simulink model "TSR_Scenario_002_cs"  (R2014b)
settings: Solver=ode5  SolverMode=SingleTasking  StartTime=0.0  StopTime=inf  FixedStep=1/100  RelTol=1e-3
PreLoadFcn:
  | mbxruntime.callbacks.PreLoadFcn(bdroot);
  | check_NUTS_defined;
  | 
  | assignin('base',['model_closed_' bdroot],false);
  | 
  | addpath('../includes_TSR/includes_TSR');
  | 
  | switch version('-release')
  | case {'2010a', '2010b', '2011a'}
  | addpath('../includes_TSR/ML2010b');
  | otherwise
  | addpath('../includes_TSR/ML2011b');
  | end
PostLoadFcn:
  | mbxruntime.callbacks.PostLoadFcn(bdroot);
InitFcn:
  | mbxruntime.callbacks.InitFcn(bdroot);;
  | 
  | addpath('..\includes_TSR');
StartFcn:
  | mbxruntime.callbacks.StartFcn(bdroot);
StopFcn:
  | mbxruntime.callbacks.StopFcn(bdroot);
model workspace: external: MAT-File .\TSR_Scenario_002_cs_hws.mat (data not in the file)
undefined symbols (not defined in the file or in its folder): InitImageOutputDir, mbxruntime, OrientationPitch, OrientationRoll, PositionX, PositionY, PositionZ, tabledata, warningInitialVelocity, x0
undefined symbols (not defined in the file): SteeringColumn, SteeringWheel, TSR_Scenario_002_cs_003e47b1b59594b6, TSR_Scenario_002_cs_023e87a31011dc74, TSR_Scenario_002_cs_048cb8409c90d9c6, TSR_Scenario_002_cs_106a0284aafa53e6, TSR_Scenario_002_cs_195b368d22a7f172, TSR_Scenario_002_cs_1e339fa5d680f213, TSR_Scenario_002_cs_26196a9fb104f950, TSR_Scenario_002_cs_261a709f6f453598, TSR_Scenario_002_cs_2ac3337370d0049d, TSR_Scenario_002_cs_2dc51e6a68b01b00, TSR_Scenario_002_cs_3460ff54d38ab2e2, TSR_Scenario_002_cs_42ea7d6e56bd6005, TSR_Scenario_002_cs_4dd419d6d2b56fc2, TSR_Scenario_002_cs_5316a21de09dff2f, TSR_Scenario_002_cs_538caacf3455966d, TSR_Scenario_002_cs_5b2cfdbcfc80811f, TSR_Scenario_002_cs_5ce0eafbb7a2dce7, TSR_Scenario_002_cs_62cdbf45c6f8824a, TSR_Scenario_002_cs_6bebc368eedff0bc, TSR_Scenario_002_cs_6d26481da4ed7e29, TSR_Scenario_002_cs_70c7e369ce6550e0, TSR_Scenario_002_cs_7a63051a1f311451, TSR_Scenario_002_cs_7d7dc8405f613c6d, TSR_Scenario_002_cs_7f65e296173485e8, TSR_Scenario_002_cs_87183cf6ff7bb4b6, TSR_Scenario_002_cs_8921b0da7ab80865, TSR_Scenario_002_cs_9495ce3a76763d1f, TSR_Scenario_002_cs_a679806a2fdc8099, TSR_Scenario_002_cs_Actros_1860_1_Path_pathUniqueID, TSR_Scenario_002_cs_Actros_2541_1_Path_pathUniqueID, TSR_Scenario_002_cs_Actros_2541_3_Path_pathUniqueID, TSR_Scenario_002_cs_Actros_2541_4_Path_pathUniqueID, TSR_Scenario_002_cs_adf24c93a9de8a4e, TSR_Scenario_002_cs_Audi_A8_1_Dynamics_Simple_initialPitch, TSR_Scenario_002_cs_Audi_A8_1_Dynamics_Simple_initialRoll, TSR_Scenario_002_cs_Audi_A8_1_Dynamics_Simple_initialX, TSR_Scenario_002_cs_Audi_A8_1_Dynamics_Simple_initialY, TSR_Scenario_002_cs_Audi_A8_1_Dynamics_Simple_initialYaw, TSR_Scenario_002_cs_Audi_A8_1_Dynamics_Simple_initialZ, TSR_Scenario_002_cs_b136c6ccb55f77db, TSR_Scenario_002_cs_ba4f809714c282b7, TSR_Scenario_002_cs_BMW_X5_1_Path_pathUniqueID, TSR_Scenario_002_cs_BMW_X5_1_SpeedProfile_speedProfileUniqueID, TSR_Scenario_002_cs_BMW_X5_2_Path_pathUniqueID, TSR_Scenario_002_cs_BMW_X5_2_SpeedProfile_speedProfileUniqueID, TSR_Scenario_002_cs_Citroen_C3_1_Path_pathUniqueID, TSR_Scenario_002_cs_Citroen_C3_2_Path_pathUniqueID, TSR_Scenario_002_cs_d8f275339b7082cf, TSR_Scenario_002_cs_Daf_95_1_Path_pathUniqueID, TSR_Scenario_002_cs_Daf_95_1_SpeedProfile_speedProfileUniqueID, TSR_Scenario_002_cs_dc019741510ce2f2, TSR_Scenario_002_cs_fdbc8aabe460b27c, TSR_Scenario_002_cs_Fiat_Bravo_1_Path_pathUniqueID, TSR_Scenario_002_cs_Ford_Fiesta_1_Path_pathUniqueID, TSR_Scenario_002_cs_Honda_Pan_European_1_Path_pathUniqueID, TSR_Scenario_002_cs_Mazda_RX8_1_Path_pathUniqueID, TSR_Scenario_002_cs_Nissan_Cabstar_1_Path_pathUniqueID, TSR_Scenario_002_cs_Nissan_Cabstar_2_Path_pathUniqueID ... (+9)
libraries: simulink_extras x82, simulink x23, PreScanSimulinkLibrary x11
(part 15 of 39)

== system TSR_Scenario_002_cs/VISUMatrixSign_HighwayOverhang_14 ==
  VISUMatrixSign_HighwayOverhang_14 : Inport  Tag=inport/VisuMatrixSign  SampleTime=1/100  BusOutputAsStruct=on
  Actuator : Subsystem  mask(PreScan Sink Block: VisuMatrixSign){UniqueID=1088, ResourceList={'1' 'InformationSign\MatrixSign_GreenArrow.png' '2' 'InformationSign\Empty.jpeg' '3' 'InformationSign\SEARCH_Logo.png' '4' 'InformationSign\z274-50_black_full.png' '5' 'InformationSign\z274-51_black_full.png' '6' 'InformationSign\z274-52_black_full.png' '7' 'InformationSign\z274-53_black_full.png' '8' 'InformationSign\z274-54_black_full.png' '9' 'InformationSign\z274-55_black_full.png' '10' 'InformationSign\z274-56_black_full.png' '11' 'InformationSign\z274-57_black_full.png' '12' 'InformationSign\z274-58_black_full.png' '13' 'InformationSign\z274-59_black_full.png' '14' 'InformationSign\z274-60_black_full.png' '15' 'InformationSign\z274-61_black_full.png' '16' 'InformationSign\z274-62_black_full.png' '17' 'InformationSign\z274-63_black_full.png' }, PivotName=}
      mask prompts: UniqueID "Parent Unique Identifier (auto-generated)"; ResourceList "Resource List (auto-generated)"; PivotName "Name of pivot (auto-generated)"
      mask help:
      | The VisuMatrixSign block provides a way to adapt the texture of the plates connected to an overhang, based on Resource IDs of the texture files.
      |
      | For more information, please click Help.
      mask Help: eval('openHelp(733)')
      mask Display: image(imread('HighwaySpeedMatrix.png'))
  wires:
  VISUMatrixSign_HighwayOverhang_14/1 -> Actuator/1(VISUMatrixSign_HighwayOverhang_14)

== system TSR_Scenario_002_cs/VISUMatrixSign_HighwayOverhang_15 ==
  VISUMatrixSign_HighwayOverhang_15 : Inport  Tag=inport/VisuMatrixSign  SampleTime=1/100  BusOutputAsStruct=on
  Actuator : Subsystem  mask(PreScan Sink Block: VisuMatrixSign){UniqueID=1090, ResourceList={'1' 'InformationSign\MatrixSign_GreenArrow.png' '2' 'InformationSign\Empty.jpeg' '3' 'InformationSign\SEARCH_Logo.png' '4' 'InformationSign\z274-50_black_full.png' '5' 'InformationSign\z274-51_black_full.png' '6' 'InformationSign\z274-52_black_full.png' '7' 'InformationSign\z274-53_black_full.png' '8' 'InformationSign\z274-54_black_full.png' '9' 'InformationSign\z274-55_black_full.png' '10' 'InformationSign\z274-56_black_full.png' '11' 'InformationSign\z274-57_black_full.png' '12' 'InformationSign\z274-58_black_full.png' '13' 'InformationSign\z274-59_black_full.png' '14' 'InformationSign\z274-60_black_full.png' '15' 'InformationSign\z274-61_black_full.png' '16' 'InformationSign\z274-62_black_full.png' '17' 'InformationSign\z274-63_black_full.png' }, PivotName=}
      mask prompts: UniqueID "Parent Unique Identifier (auto-generated)"; ResourceList "Resource List (auto-generated)"; PivotName "Name of pivot (auto-generated)"
      mask help:
      | The VisuMatrixSign block provides a way to adapt the texture of the plates connected to an overhang, based on Resource IDs of the texture files.
      |
      | For more information, please click Help.
      mask Help: eval('openHelp(733)')
      mask Display: image(imread('HighwaySpeedMatrix.png'))
  wires:
  VISUMatrixSign_HighwayOverhang_15/1 -> Actuator/1(VISUMatrixSign_HighwayOverhang_15)

== system TSR_Scenario_002_cs/VISUMatrixSign_HighwayOverhang_16 ==
  VISUMatrixSign_HighwayOverhang_16 : Inport  Tag=inport/VisuMatrixSign  SampleTime=1/100  BusOutputAsStruct=on
  Actuator : Subsystem  mask(PreScan Sink Block: VisuMatrixSign){UniqueID=1091, ResourceList={'1' 'InformationSign\MatrixSign_GreenArrow.png' '2' 'InformationSign\Empty.jpeg' '3' 'InformationSign\SEARCH_Logo.png' '4' 'InformationSign\z274-50_black_full.png' '5' 'InformationSign\z274-51_black_full.png' '6' 'InformationSign\z274-52_black_full.png' '7' 'InformationSign\z274-53_black_full.png' '8' 'InformationSign\z274-54_black_full.png' '9' 'InformationSign\z274-55_black_full.png' '10' 'InformationSign\z274-56_black_full.png' '11' 'InformationSign\z274-57_black_full.png' '12' 'InformationSign\z274-58_black_full.png' '13' 'InformationSign\z274-59_black_full.png' '14' 'InformationSign\z274-60_black_full.png' '15' 'InformationSign\z274-61_black_full.png' '16' 'InformationSign\z274-62_black_full.png' '17' 'InformationSign\z274-63_black_full.png' }, PivotName=}
      mask prompts: UniqueID "Parent Unique Identifier (auto-generated)"; ResourceList "Resource List (auto-generated)"; PivotName "Name of pivot (auto-generated)"
      mask help:
      | The VisuMatrixSign block provides a way to adapt the texture of the plates connected to an overhang, based on Resource IDs of the texture files.
      |
      | For more information, please click Help.
      mask Help: eval('openHelp(733)')
      mask Display: image(imread('HighwaySpeedMatrix.png'))
  wires:
  VISUMatrixSign_HighwayOverhang_16/1 -> Actuator/1(VISUMatrixSign_HighwayOverhang_16)

== system TSR_Scenario_002_cs/VISUMatrixSign_HighwayOverhang_17 ==
  VISUMatrixSign_HighwayOverhang_17 : Inport  Tag=inport/VisuMatrixSign  SampleTime=1/100  BusOutputAsStruct=on
  Actuator : Subsystem  mask(PreScan Sink Block: VisuMatrixSign){UniqueID=1092, ResourceList={'1' 'InformationSign\MatrixSign_GreenArrow.png' '2' 'InformationSign\Empty.jpeg' '3' 'InformationSign\SEARCH_Logo.png' '4' 'InformationSign\z274-50_black_full.png' '5' 'InformationSign\z274-51_black_full.png' '6' 'InformationSign\z274-52_black_full.png' '7' 'InformationSign\z274-53_black_full.png' '8' 'InformationSign\z274-54_black_full.png' '9' 'InformationSign\z274-55_black_full.png' '10' 'InformationSign\z274-56_black_full.png' '11' 'InformationSign\z274-57_black_full.png' '12' 'InformationSign\z274-58_black_full.png' '13' 'InformationSign\z274-59_black_full.png' '14' 'InformationSign\z274-60_black_full.png' '15' 'InformationSign\z274-61_black_full.png' '16' 'InformationSign\z274-62_black_full.png' '17' 'InformationSign\z274-63_black_full.png' }, PivotName=}
      mask prompts: UniqueID "Parent Unique Identifier (auto-generated)"; ResourceList "Resource List (auto-generated)"; PivotName "Name of pivot (auto-generated)"
      mask help:
      | The VisuMatrixSign block provides a way to adapt the texture of the plates connected to an overhang, based on Resource IDs of the texture files.
      |
      | For more information, please click Help.
      mask Help: eval('openHelp(733)')
      mask Display: image(imread('HighwaySpeedMatrix.png'))
  wires:
  VISUMatrixSign_HighwayOverhang_17/1 -> Actuator/1(VISUMatrixSign_HighwayOverhang_17)

== system TSR_Scenario_002_cs/VISUMatrixSign_HighwayOverhang_18 ==
  VISUMatrixSign_HighwayOverhang_18 : Inport  Tag=inport/VisuMatrixSign  SampleTime=1/100  BusOutputAsStruct=on
  Actuator : Subsystem  mask(PreScan Sink Block: VisuMatrixSign){UniqueID=1093, ResourceList={'1' 'InformationSign\MatrixSign_GreenArrow.png' '2' 'InformationSign\Empty.jpeg' '3' 'InformationSign\SEARCH_Logo.png' '4' 'InformationSign\z274-50_black_full.png' '5' 'InformationSign\z274-51_black_full.png' '6' 'InformationSign\z274-52_black_full.png' '7' 'InformationSign\z274-53_black_full.png' '8' 'InformationSign\z274-54_black_full.png' '9' 'InformationSign\z274-55_black_full.png' '10' 'InformationSign\z274-56_black_full.png' '11' 'InformationSign\z274-57_black_full.png' '12' 'InformationSign\z274-58_black_full.png' '13' 'InformationSign\z274-59_black_full.png' '14' 'InformationSign\z274-60_black_full.png' '15' 'InformationSign\z274-61_black_full.png' '16' 'InformationSign\z274-62_black_full.png' '17' 'InformationSign\z274-63_black_full.png' }, PivotName=}
      mask prompts: UniqueID "Parent Unique Identifier (auto-generated)"; ResourceList "Resource List (auto-generated)"; PivotName "Name of pivot (auto-generated)"
      mask help:
      | The VisuMatrixSign block provides a way to adapt the texture of the plates connected to an overhang, based on Resource IDs of the texture files.
      |
      | For more information, please click Help.
      mask Help: eval('openHelp(733)')
      mask Display: image(imread('HighwaySpeedMatrix.png'))
  wires:
  VISUMatrixSign_HighwayOverhang_18/1 -> Actuator/1(VISUMatrixSign_HighwayOverhang_18)

== system TSR_Scenario_002_cs/VISUMatrixSign_HighwayOverhang_19 ==
  VISUMatrixSign_HighwayOverhang_19 : Inport  Tag=inport/VisuMatrixSign  SampleTime=1/100  BusOutputAsStruct=on
  Actuator : Subsystem  mask(PreScan Sink Block: VisuMatrixSign){UniqueID=1095, ResourceList={'1' 'InformationSign\MatrixSign_GreenArrow.png' '2' 'InformationSign\Empty.jpeg' '3' 'InformationSign\SEARCH_Logo.png' '4' 'InformationSign\z274-50_black_full.png' '5' 'InformationSign\z274-51_black_full.png' '6' 'InformationSign\z274-52_black_full.png' '7' 'InformationSign\z274-53_black_full.png' '8' 'InformationSign\z274-54_black_full.png' '9' 'InformationSign\z274-55_black_full.png' '10' 'InformationSign\z274-56_black_full.png' '11' 'InformationSign\z274-57_black_full.png' '12' 'InformationSign\z274-58_black_full.png' '13' 'InformationSign\z274-59_black_full.png' '14' 'InformationSign\z274-60_black_full.png' '15' 'InformationSign\z274-61_black_full.png' '16' 'InformationSign\z274-62_black_full.png' '17' 'InformationSign\z274-63_black_full.png' }, PivotName=}
      mask prompts: UniqueID "Parent Unique Identifier (auto-generated)"; ResourceList "Resource List (auto-generated)"; PivotName "Name of pivot (auto-generated)"
      mask help:
      | The VisuMatrixSign block provides a way to adapt the texture of the plates connected to an overhang, based on Resource IDs of the texture files.
      |
      | For more information, please click Help.
      mask Help: eval('openHelp(733)')
      mask Display: image(imread('HighwaySpeedMatrix.png'))
  wires:
  VISUMatrixSign_HighwayOverhang_19/1 -> Actuator/1(VISUMatrixSign_HighwayOverhang_19)

== system TSR_Scenario_002_cs/VISUMatrixSign_HighwayOverhang_2 ==
  VISUMatrixSign_HighwayOverhang_2 : Inport  Tag=inport/VisuMatrixSign  SampleTime=1/100  BusOutputAsStruct=on
  Actuator : Subsystem  mask(PreScan Sink Block: VisuMatrixSign){UniqueID=432, ResourceList={'1' 'InformationSign\MatrixSign_GreenArrow.png' '2' 'InformationSign\Empty.jpeg' '3' 'InformationSign\SEARCH_Logo.png' '4' 'InformationSign\z274-50_black_full.png' '5' 'InformationSign\z274-51_black_full.png' '6' 'InformationSign\z274-52_black_full.png' '7' 'InformationSign\z274-53_black_full.png' '8' 'InformationSign\z274-54_black_full.png' '9' 'InformationSign\z274-55_black_full.png' '10' 'InformationSign\z274-56_black_full.png' '11' 'InformationSign\z274-57_black_full.png' '12' 'InformationSign\z274-58_black_full.png' '13' 'InformationSign\z274-59_black_full.png' '14' 'InformationSign\z274-60_black_full.png' '15' 'InformationSign\z274-61_black_full.png' '16' 'InformationSign\z274-62_black_full.png' '17' 'InformationSign\z274-63_black_full.png' }, PivotName=}
      mask prompts: UniqueID "Parent Unique Identifier (auto-generated)"; ResourceList "Resource List (auto-generated)"; PivotName "Name of pivot (auto-generated)"
      mask help:
      | The VisuMatrixSign block provides a way to adapt the texture of the plates connected to an overhang, based on Resource IDs of the texture files.
      |
      | For more information, please click Help.
      mask Help: eval('openHelp(733)')
      mask Display: image(imread('HighwaySpeedMatrix.png'))
  wires:
  VISUMatrixSign_HighwayOverhang_2/1 -> Actuator/1(VISUMatrixSign_HighwayOverhang_2)

== system TSR_Scenario_002_cs/VISUMatrixSign_HighwayOverhang_20 ==
  VISUMatrixSign_HighwayOverhang_20 : Inport  Tag=inport/VisuMatrixSign  SampleTime=1/100  BusOutputAsStruct=on
  Actuator : Subsystem  mask(PreScan Sink Block: VisuMatrixSign){UniqueID=1094, ResourceList={'1' 'InformationSign\MatrixSign_GreenArrow.png' '2' 'InformationSign\Empty.jpeg' '3' 'InformationSign\SEARCH_Logo.png' '4' 'InformationSign\z274-50_black_full.png' '5' 'InformationSign\z274-51_black_full.png' '6' 'InformationSign\z274-52_black_full.png' '7' 'InformationSign\z274-53_black_full.png' '8' 'InformationSign\z274-54_black_full.png' '9' 'InformationSign\z274-55_black_full.png' '10' 'InformationSign\z274-56_black_full.png' '11' 'InformationSign\z274-57_black_full.png' '12' 'InformationSign\z274-58_black_full.png' '13' 'InformationSign\z274-59_black_full.png' '14' 'InformationSign\z274-60_black_full.png' '15' 'InformationSign\z274-61_black_full.png' '16' 'InformationSign\z274-62_black_full.png' '17' 'InformationSign\z274-63_black_full.png' }, PivotName=}
      mask prompts: UniqueID "Parent Unique Identifier (auto-generated)"; ResourceList "Resource List (auto-generated)"; PivotName "Name of pivot (auto-generated)"
      mask help:
      | The VisuMatrixSign block provides a way to adapt the texture of the plates connected to an overhang, based on Resource IDs of the texture files.
      |
      | For more information, please click Help.
      mask Help: eval('openHelp(733)')
      mask Display: image(imread('HighwaySpeedMatrix.png'))
  wires:
  VISUMatrixSign_HighwayOverhang_20/1 -> Actuator/1(VISUMatrixSign_HighwayOverhang_20)

== system TSR_Scenario_002_cs/VISUMatrixSign_HighwayOverhang_21 ==
  VISUMatrixSign_HighwayOverhang_21 : Inport  Tag=inport/VisuMatrixSign  SampleTime=1/100  BusOutputAsStruct=on
  Actuator : Subsystem  mask(PreScan Sink Block: VisuMatrixSign){UniqueID=1099, ResourceList={'1' 'InformationSign\MatrixSign_GreenArrow.png' '2' 'InformationSign\Empty.jpeg' '3' 'InformationSign\SEARCH_Logo.png' '4' 'InformationSign\z274-50_black_full.png' '5' 'InformationSign\z274-51_black_full.png' '6' 'InformationSign\z274-52_black_full.png' '7' 'InformationSign\z274-53_black_full.png' '8' 'InformationSign\z274-54_black_full.png' '9' 'InformationSign\z274-55_black_full.png' '10' 'InformationSign\z274-56_black_full.png' '11' 'InformationSign\z274-57_black_full.png' '12' 'InformationSign\z274-58_black_full.png' '13' 'InformationSign\z274-59_black_full.png' '14' 'InformationSign\z274-60_black_full.png' '15' 'InformationSign\z274-61_black_full.png' '16' 'InformationSign\z274-62_black_full.png' '17' 'InformationSign\z274-63_black_full.png' }, PivotName=}
      mask prompts: UniqueID "Parent Unique Identifier (auto-generated)"; ResourceList "Resource List (auto-generated)"; PivotName "Name of pivot (auto-generated)"
      mask help:
      | The VisuMatrixSign block provides a way to adapt the texture of the plates connected to an overhang, based on Resource IDs of the texture files.
      |
      | For more information, please click Help.
      mask Help: eval('openHelp(733)')
      mask Display: image(imread('HighwaySpeedMatrix.png'))
  wires:
  VISUMatrixSign_HighwayOverhang_21/1 -> Actuator/1(VISUMatrixSign_HighwayOverhang_21)

== system TSR_Scenario_002_cs/VISUMatrixSign_HighwayOverhang_22 ==
  VISUMatrixSign_HighwayOverhang_22 : Inport  Tag=inport/VisuMatrixSign  SampleTime=1/100  BusOutputAsStruct=on
  Actuator : Subsystem  mask(PreScan Sink Block: VisuMatrixSign){UniqueID=1100, ResourceList={'1' 'InformationSign\MatrixSign_GreenArrow.png' '2' 'InformationSign\Empty.jpeg' '3' 'InformationSign\SEARCH_Logo.png' '4' 'InformationSign\z274-50_black_full.png' '5' 'InformationSign\z274-51_black_full.png' '6' 'InformationSign\z274-52_black_full.png' '7' 'InformationSign\z274-53_black_full.png' '8' 'InformationSign\z274-54_black_full.png' '9' 'InformationSign\z274-55_black_full.png' '10' 'InformationSign\z274-56_black_full.png' '11' 'InformationSign\z274-57_black_full.png' '12' 'InformationSign\z274-58_black_full.png' '13' 'InformationSign\z274-59_black_full.png' '14' 'InformationSign\z274-60_black_full.png' '15' 'InformationSign\z274-61_black_full.png' '16' 'InformationSign\z274-62_black_full.png' '17' 'InformationSign\z274-63_black_full.png' }, PivotName=}
      mask prompts: UniqueID "Parent Unique Identifier (auto-generated)"; ResourceList "Resource List (auto-generated)"; PivotName "Name of pivot (auto-generated)"
      mask help:
      | The VisuMatrixSign block provides a way to adapt the texture of the plates connected to an overhang, based on Resource IDs of the texture files.
      |
      | For more information, please click Help.
      mask Help: eval('openHelp(733)')
      mask Display: image(imread('HighwaySpeedMatrix.png'))
  wires:
  VISUMatrixSign_HighwayOverhang_22/1 -> Actuator/1(VISUMatrixSign_HighwayOverhang_22)

== system TSR_Scenario_002_cs/VISUMatrixSign_HighwayOverhang_23 ==
  VISUMatrixSign_HighwayOverhang_23 : Inport  Tag=inport/VisuMatrixSign  SampleTime=1/100  BusOutputAsStruct=on
  Actuator : Subsystem  mask(PreScan Sink Block: VisuMatrixSign){UniqueID=1102, ResourceList={'1' 'InformationSign\MatrixSign_GreenArrow.png' '2' 'InformationSign\Empty.jpeg' '3' 'InformationSign\SEARCH_Logo.png' '4' 'InformationSign\z274-50_black_full.png' '5' 'InformationSign\z274-51_black_full.png' '6' 'InformationSign\z274-52_black_full.png' '7' 'InformationSign\z274-53_black_full.png' '8' 'InformationSign\z274-54_black_full.png' '9' 'InformationSign\z274-55_black_full.png' '10' 'InformationSign\z274-56_black_full.png' '11' 'InformationSign\z274-57_black_full.png' '12' 'InformationSign\z274-58_black_full.png' '13' 'InformationSign\z274-59_black_full.png' '14' 'InformationSign\z274-60_black_full.png' '15' 'InformationSign\z274-61_black_full.png' '16' 'InformationSign\z274-62_black_full.png' '17' 'InformationSign\z274-63_black_full.png' }, PivotName=}
      mask prompts: UniqueID "Parent Unique Identifier (auto-generated)"; ResourceList "Resource List (auto-generated)"; PivotName "Name of pivot (auto-generated)"
      mask help:
      | The VisuMatrixSign block provides a way to adapt the texture of the plates connected to an overhang, based on Resource IDs of the texture files.
      |
      | For more information, please click Help.
      mask Help: eval('openHelp(733)')
      mask Display: image(imread('HighwaySpeedMatrix.png'))
  wires:
  VISUMatrixSign_HighwayOverhang_23/1 -> Actuator/1(VISUMatrixSign_HighwayOverhang_23)

== system TSR_Scenario_002_cs/VISUMatrixSign_HighwayOverhang_24 ==
  VISUMatrixSign_HighwayOverhang_24 : Inport  Tag=inport/VisuMatrixSign  SampleTime=1/100  BusOutputAsStruct=on
  Actuator : Subsystem  mask(PreScan Sink Block: VisuMatrixSign){UniqueID=1103, ResourceList={'1' 'InformationSign\MatrixSign_GreenArrow.png' '2' 'InformationSign\Empty.jpeg' '3' 'InformationSign\SEARCH_Logo.png' '4' 'InformationSign\z274-50_black_full.png' '5' 'InformationSign\z274-51_black_full.png' '6' 'InformationSign\z274-52_black_full.png' '7' 'InformationSign\z274-53_black_full.png' '8' 'InformationSign\z274-54_black_full.png' '9' 'InformationSign\z274-55_black_full.png' '10' 'InformationSign\z274-56_black_full.png' '11' 'InformationSign\z274-57_black_full.png' '12' 'InformationSign\z274-58_black_full.png' '13' 'InformationSign\z274-59_black_full.png' '14' 'InformationSign\z274-60_black_full.png' '15' 'InformationSign\z274-61_black_full.png' '16' 'InformationSign\z274-62_black_full.png' '17' 'InformationSign\z274-63_black_full.png' }, PivotName=}
      mask prompts: UniqueID "Parent Unique Identifier (auto-generated)"; ResourceList "Resource List (auto-generated)"; PivotName "Name of pivot (auto-generated)"
      mask help:
      | The VisuMatrixSign block provides a way to adapt the texture of the plates connected to an overhang, based on Resource IDs of the texture files.
      |
      | For more information, please click Help.
      mask Help: eval('openHelp(733)')
      mask Display: image(imread('HighwaySpeedMatrix.png'))
  wires:
  VISUMatrixSign_HighwayOverhang_24/1 -> Actuator/1(VISUMatrixSign_HighwayOverhang_24)

== system TSR_Scenario_002_cs/VISUMatrixSign_HighwayOverhang_25 ==
  VISUMatrixSign_HighwayOverhang_25 : Inport  Tag=inport/VisuMatrixSign  SampleTime=1/100  BusOutputAsStruct=on
  Actuator : Subsystem  mask(PreScan Sink Block: VisuMatrixSign){UniqueID=1104, ResourceList={'1' 'InformationSign\MatrixSign_GreenArrow.png' '2' 'InformationSign\Empty.jpeg' '3' 'InformationSign\SEARCH_Logo.png' '4' 'InformationSign\z274-50_black_full.png' '5' 'InformationSign\z274-51_black_full.png' '6' 'InformationSign\z274-52_black_full.png' '7' 'InformationSign\z274-53_black_full.png' '8' 'InformationSign\z274-54_black_full.png' '9' 'InformationSign\z274-55_black_full.png' '10' 'InformationSign\z274-56_black_full.png' '11' 'InformationSign\z274-57_black_full.png' '12' 'InformationSign\z274-58_black_full.png' '13' 'InformationSign\z274-59_black_full.png' '14' 'InformationSign\z274-60_black_full.png' '15' 'InformationSign\z274-61_black_full.png' '16' 'InformationSign\z274-62_black_full.png' '17' 'InformationSign\z274-63_black_full.png' }, PivotName=}
      mask prompts: UniqueID "Parent Unique Identifier (auto-generated)"; ResourceList "Resource List (auto-generated)"; PivotName "Name of pivot (auto-generated)"
      mask help:
      | The VisuMatrixSign block provides a way to adapt the texture of the plates connected to an overhang, based on Resource IDs of the texture files.
      |
      | For more information, please click Help.
      mask Help: eval('openHelp(733)')
      mask Display: image(imread('HighwaySpeedMatrix.png'))
  wires:
  VISUMatrixSign_HighwayOverhang_25/1 -> Actuator/1(VISUMatrixSign_HighwayOverhang_25)

== system TSR_Scenario_002_cs/VISUMatrixSign_HighwayOverhang_26 ==
  VISUMatrixSign_HighwayOverhang_26 : Inport  Tag=inport/VisuMatrixSign  SampleTime=1/100  BusOutputAsStruct=on
  Actuator : Subsystem  mask(PreScan Sink Block: VisuMatrixSign){UniqueID=1105, ResourceList={'1' 'InformationSign\MatrixSign_GreenArrow.png' '2' 'InformationSign\Empty.jpeg' '3' 'InformationSign\SEARCH_Logo.png' '4' 'InformationSign\z274-50_black_full.png' '5' 'InformationSign\z274-51_black_full.png' '6' 'InformationSign\z274-52_black_full.png' '7' 'InformationSign\z274-53_black_full.png' '8' 'InformationSign\z274-54_black_full.png' '9' 'InformationSign\z274-55_black_full.png' '10' 'InformationSign\z274-56_black_full.png' '11' 'InformationSign\z274-57_black_full.png' '12' 'InformationSign\z274-58_black_full.png' '13' 'InformationSign\z274-59_black_full.png' '14' 'InformationSign\z274-60_black_full.png' '15' 'InformationSign\z274-61_black_full.png' '16' 'InformationSign\z274-62_black_full.png' '17' 'InformationSign\z274-63_black_full.png' }, PivotName=}
      mask prompts: UniqueID "Parent Unique Identifier (auto-generated)"; ResourceList "Resource List (auto-generated)"; PivotName "Name of pivot (auto-generated)"
      mask help:
      | The VisuMatrixSign block provides a way to adapt the texture of the plates connected to an overhang, based on Resource IDs of the texture files.
      |
      | For more information, please click Help.
      mask Help: eval('openHelp(733)')
      mask Display: image(imread('HighwaySpeedMatrix.png'))
  wires:
  VISUMatrixSign_HighwayOverhang_26/1 -> Actuator/1(VISUMatrixSign_HighwayOverhang_26)

== system TSR_Scenario_002_cs/VISUMatrixSign_HighwayOverhang_27 ==
  VISUMatrixSign_HighwayOverhang_27 : Inport  Tag=inport/VisuMatrixSign  SampleTime=1/100  BusOutputAsStruct=on
  Actuator : Subsystem  mask(PreScan Sink Block: VisuMatrixSign){UniqueID=1106, ResourceList={'1' 'InformationSign\MatrixSign_GreenArrow.png' '2' 'InformationSign\Empty.jpeg' '3' 'InformationSign\SEARCH_Logo.png' '4' 'InformationSign\z274-50_black_full.png' '5' 'InformationSign\z274-51_black_full.png' '6' 'InformationSign\z274-52_black_full.png' '7' 'InformationSign\z274-53_black_full.png' '8' 'InformationSign\z274-54_black_full.png' '9' 'InformationSign\z274-55_black_full.png' '10' 'InformationSign\z274-56_black_full.png' '11' 'InformationSign\z274-57_black_full.png' '12' 'InformationSign\z274-58_black_full.png' '13' 'InformationSign\z274-59_black_full.png' '14' 'InformationSign\z274-60_black_full.png' '15' 'InformationSign\z274-61_black_full.png' '16' 'InformationSign\z274-62_black_full.png' '17' 'InformationSign\z274-63_black_full.png' }, PivotName=}
      mask prompts: UniqueID "Parent Unique Identifier (auto-generated)"; ResourceList "Resource List (auto-generated)"; PivotName "Name of pivot (auto-generated)"
      mask help:
      | The VisuMatrixSign block provides a way to adapt the texture of the plates connected to an overhang, based on Resource IDs of the texture files.
      |
      | For more information, please click Help.
      mask Help: eval('openHelp(733)')
      mask Display: image(imread('HighwaySpeedMatrix.png'))
  wires:
  VISUMatrixSign_HighwayOverhang_27/1 -> Actuator/1(VISUMatrixSign_HighwayOverhang_27)

== system TSR_Scenario_002_cs/VISUMatrixSign_HighwayOverhang_28 ==
  VISUMatrixSign_HighwayOverhang_28 : Inport  Tag=inport/VisuMatrixSign  SampleTime=1/100  BusOutputAsStruct=on
  Actuator : Subsystem  mask(PreScan Sink Block: VisuMatrixSign){UniqueID=1107, ResourceList={'1' 'InformationSign\MatrixSign_GreenArrow.png' '2' 'InformationSign\Empty.jpeg' '3' 'InformationSign\SEARCH_Logo.png' '4' 'InformationSign\z274-50_black_full.png' '5' 'InformationSign\z274-51_black_full.png' '6' 'InformationSign\z274-52_black_full.png' '7' 'InformationSign\z274-53_black_full.png' '8' 'InformationSign\z274-54_black_full.png' '9' 'InformationSign\z274-55_black_full.png' '10' 'InformationSign\z274-56_black_full.png' '11' 'InformationSign\z274-57_black_full.png' '12' 'InformationSign\z274-58_black_full.png' '13' 'InformationSign\z274-59_black_full.png' '14' 'InformationSign\z274-60_black_full.png' '15' 'InformationSign\z274-61_black_full.png' '16' 'InformationSign\z274-62_black_full.png' '17' 'InformationSign\z274-63_black_full.png' }, PivotName=}
      mask prompts: UniqueID "Parent Unique Identifier (auto-generated)"; ResourceList "Resource List (auto-generated)"; PivotName "Name of pivot (auto-generated)"
      mask help:
      | The VisuMatrixSign block provides a way to adapt the texture of the plates connected to an overhang, based on Resource IDs of the texture files.
      |
      | For more information, please click Help.
      mask Help: eval('openHelp(733)')
      mask Display: image(imread('HighwaySpeedMatrix.png'))
  wires:
  VISUMatrixSign_HighwayOverhang_28/1 -> Actuator/1(VISUMatrixSign_HighwayOverhang_28)

== system TSR_Scenario_002_cs/VISUMatrixSign_HighwayOverhang_3 ==
  VISUMatrixSign_HighwayOverhang_3 : Inport  Tag=inport/VisuMatrixSign  SampleTime=1/100  BusOutputAsStruct=on
  Actuator : Subsystem  mask(PreScan Sink Block: VisuMatrixSign){UniqueID=440, ResourceList={'1' 'InformationSign\MatrixSign_GreenArrow.png' '2' 'InformationSign\Empty.jpeg' '3' 'InformationSign\SEARCH_Logo.png' '4' 'InformationSign\z274-50_black_full.png' '5' 'InformationSign\z274-51_black_full.png' '6' 'InformationSign\z274-52_black_full.png' '7' 'InformationSign\z274-53_black_full.png' '8' 'InformationSign\z274-54_black_full.png' '9' 'InformationSign\z274-55_black_full.png' '10' 'InformationSign\z274-56_black_full.png' '11' 'InformationSign\z274-57_black_full.png' '12' 'InformationSign\z274-58_black_full.png' '13' 'InformationSign\z274-59_black_full.png' '14' 'InformationSign\z274-60_black_full.png' '15' 'InformationSign\z274-61_black_full.png' '16' 'InformationSign\z274-62_black_full.png' '17' 'InformationSign\z274-63_black_full.png' }, PivotName=}
      mask prompts: UniqueID "Parent Unique Identifier (auto-generated)"; ResourceList "Resource List (auto-generated)"; PivotName "Name of pivot (auto-generated)"
      mask help:
      | The VisuMatrixSign block provides a way to adapt the texture of the plates connected to an overhang, based on Resource IDs of the texture files.
      |
      | For more information, please click Help.
      mask Help: eval('openHelp(733)')
      mask Display: image(imread('HighwaySpeedMatrix.png'))
  wires:
  VISUMatrixSign_HighwayOverhang_3/1 -> Actuator/1(VISUMatrixSign_HighwayOverhang_3)

== system TSR_Scenario_002_cs/VISUMatrixSign_HighwayOverhang_4 ==
  VISUMatrixSign_HighwayOverhang_4 : Inport  Tag=inport/VisuMatrixSign  SampleTime=1/100  BusOutputAsStruct=on
  Actuator : Subsystem  mask(PreScan Sink Block: VisuMatrixSign){UniqueID=441, ResourceList={'1' 'InformationSign\MatrixSign_GreenArrow.png' '2' 'InformationSign\Empty.jpeg' '3' 'InformationSign\SEARCH_Logo.png' '4' 'InformationSign\z274-50_black_full.png' '5' 'InformationSign\z274-51_black_full.png' '6' 'InformationSign\z274-52_black_full.png' '7' 'InformationSign\z274-53_black_full.png' '8' 'InformationSign\z274-54_black_full.png' '9' 'InformationSign\z274-55_black_full.png' '10' 'InformationSign\z274-56_black_full.png' '11' 'InformationSign\z274-57_black_full.png' '12' 'InformationSign\z274-58_black_full.png' '13' 'InformationSign\z274-59_black_full.png' '14' 'InformationSign\z274-60_black_full.png' '15' 'InformationSign\z274-61_black_full.png' '16' 'InformationSign\z274-62_black_full.png' '17' 'InformationSign\z274-63_black_full.png' }, PivotName=}
      mask prompts: UniqueID "Parent Unique Identifier (auto-generated)"; ResourceList "Resource List (auto-generated)"; PivotName "Name of pivot (auto-generated)"
      mask help:
      | The VisuMatrixSign block provides a way to adapt the texture of the plates connected to an overhang, based on Resource IDs of the texture files.
      |
      | For more information, please click Help.
      mask Help: eval('openHelp(733)')
      mask Display: image(imread('HighwaySpeedMatrix.png'))
  wires:
  VISUMatrixSign_HighwayOverhang_4/1 -> Actuator/1(VISUMatrixSign_HighwayOverhang_4)

== system TSR_Scenario_002_cs/VISUMatrixSign_HighwayOverhang_5 ==
  VISUMatrixSign_HighwayOverhang_5 : Inport  Tag=inport/VisuMatrixSign  SampleTime=1/100  BusOutputAsStruct=on
  Actuator : Subsystem  mask(PreScan Sink Block: VisuMatrixSign){UniqueID=843, ResourceList={'1' 'InformationSign\MatrixSign_GreenArrow.png' '2' 'InformationSign\Empty.jpeg' '3' 'InformationSign\SEARCH_Logo.png' '4' 'InformationSign\z274-50_black_full.png' '5' 'InformationSign\z274-51_black_full.png' '6' 'InformationSign\z274-52_black_full.png' '7' 'InformationSign\z274-53_black_full.png' '8' 'InformationSign\z274-54_black_full.png' '9' 'InformationSign\z274-55_black_full.png' '10' 'InformationSign\z274-56_black_full.png' '11' 'InformationSign\z274-57_black_full.png' '12' 'InformationSign\z274-58_black_full.png' '13' 'InformationSign\z274-59_black_full.png' '14' 'InformationSign\z274-60_black_full.png' '15' 'InformationSign\z274-61_black_full.png' '16' 'InformationSign\z274-62_black_full.png' '17' 'InformationSign\z274-63_black_full.png' }, PivotName=}
      mask prompts: UniqueID "Parent Unique Identifier (auto-generated)"; ResourceList "Resource List (auto-generated)"; PivotName "Name of pivot (auto-generated)"
      mask help:
      | The VisuMatrixSign block provides a way to adapt the texture of the plates connected to an overhang, based on Resource IDs of the texture files.
      |
      | For more information, please click Help.
      mask Help: eval('openHelp(733)')
      mask Display: image(imread('HighwaySpeedMatrix.png'))
  wires:
  VISUMatrixSign_HighwayOverhang_5/1 -> Actuator/1(VISUMatrixSign_HighwayOverhang_5)

== system TSR_Scenario_002_cs/VISUMatrixSign_HighwayOverhang_6 ==
  VISUMatrixSign_HighwayOverhang_6 : Inport  Tag=inport/VisuMatrixSign  SampleTime=1/100  BusOutputAsStruct=on
  Actuator : Subsystem  mask(PreScan Sink Block: VisuMatrixSign){UniqueID=846, ResourceList={'1' 'InformationSign\MatrixSign_GreenArrow.png' '2' 'InformationSign\Empty.jpeg' '3' 'InformationSign\SEARCH_Logo.png' '4' 'InformationSign\z274-50_black_full.png' '5' 'InformationSign\z274-51_black_full.png' '6' 'InformationSign\z274-52_black_full.png' '7' 'InformationSign\z274-53_black_full.png' '8' 'InformationSign\z274-54_black_full.png' '9' 'InformationSign\z274-55_black_full.png' '10' 'InformationSign\z274-56_black_full.png' '11' 'InformationSign\z274-57_black_full.png' '12' 'InformationSign\z274-58_black_full.png' '13' 'InformationSign\z274-59_black_full.png' '14' 'InformationSign\z274-60_black_full.png' '15' 'InformationSign\z274-61_black_full.png' '16' 'InformationSign\z274-62_black_full.png' '17' 'InformationSign\z274-63_black_full.png' }, PivotName=}
      mask prompts: UniqueID "Parent Unique Identifier (auto-generated)"; ResourceList "Resource List (auto-generated)"; PivotName "Name of pivot (auto-generated)"
      mask help:
      | The VisuMatrixSign block provides a way to adapt the texture of the plates connected to an overhang, based on Resource IDs of the texture files.
      |
      | For more information, please click Help.
      mask Help: eval('openHelp(733)')
      mask Display: image(imread('HighwaySpeedMatrix.png'))
  wires:
  VISUMatrixSign_HighwayOverhang_6/1 -> Actuator/1(VISUMatrixSign_HighwayOverhang_6)

== system TSR_Scenario_002_cs/VISUMatrixSign_HighwayOverhang_7 ==
  VISUMatrixSign_HighwayOverhang_7 : Inport  Tag=inport/VisuMatrixSign  SampleTime=1/100  BusOutputAsStruct=on
  Actuator : Subsystem  mask(PreScan Sink Block: VisuMatrixSign){UniqueID=867, ResourceList={'1' 'InformationSign\MatrixSign_GreenArrow.png' '2' 'InformationSign\Empty.jpeg' '3' 'InformationSign\SEARCH_Logo.png' '4' 'InformationSign\z274-50_black_full.png' '5' 'InformationSign\z274-51_black_full.png' '6' 'InformationSign\z274-52_black_full.png' '7' 'InformationSign\z274-53_black_full.png' '8' 'InformationSign\z274-54_black_full.png' '9' 'InformationSign\z274-55_black_full.png' '10' 'InformationSign\z274-56_black_full.png' '11' 'InformationSign\z274-57_black_full.png' '12' 'InformationSign\z274-58_black_full.png' '13' 'InformationSign\z274-59_black_full.png' '14' 'InformationSign\z274-60_black_full.png' '15' 'InformationSign\z274-61_black_full.png' '16' 'InformationSign\z274-62_black_full.png' '17' 'InformationSign\z274-63_black_full.png' }, PivotName=}
      mask prompts: UniqueID "Parent Unique Identifier (auto-generated)"; ResourceList "Resource List (auto-generated)"; PivotName "Name of pivot (auto-generated)"
      mask help:
      | The VisuMatrixSign block provides a way to adapt the texture of the plates connected to an overhang, based on Resource IDs of the texture files.
      |
      | For more information, please click Help.
      mask Help: eval('openHelp(733)')
      mask Display: image(imread('HighwaySpeedMatrix.png'))
  wires:
  VISUMatrixSign_HighwayOverhang_7/1 -> Actuator/1(VISUMatrixSign_HighwayOverhang_7)

== system TSR_Scenario_002_cs/VISUMatrixSign_HighwayOverhang_8 ==
  VISUMatrixSign_HighwayOverhang_8 : Inport  Tag=inport/VisuMatrixSign  SampleTime=1/100  BusOutputAsStruct=on
  Actuator : Subsystem  mask(PreScan Sink Block: VisuMatrixSign){UniqueID=870, ResourceList={'1' 'InformationSign\MatrixSign_GreenArrow.png' '2' 'InformationSign\Empty.jpeg' '3' 'InformationSign\SEARCH_Logo.png' '4' 'InformationSign\z274-50_black_full.png' '5' 'InformationSign\z274-51_black_full.png' '6' 'InformationSign\z274-52_black_full.png' '7' 'InformationSign\z274-53_black_full.png' '8' 'InformationSign\z274-54_black_full.png' '9' 'InformationSign\z274-55_black_full.png' '10' 'InformationSign\z274-56_black_full.png' '11' 'InformationSign\z274-57_black_full.png' '12' 'InformationSign\z274-58_black_full.png' '13' 'InformationSign\z274-59_black_full.png' '14' 'InformationSign\z274-60_black_full.png' '15' 'InformationSign\z274-61_black_full.png' '16' 'InformationSign\z274-62_black_full.png' '17' 'InformationSign\z274-63_black_full.png' }, PivotName=}
      mask prompts: UniqueID "Parent Unique Identifier (auto-generated)"; ResourceList "Resource List (auto-generated)"; PivotName "Name of pivot (auto-generated)"
      mask help:
      | The VisuMatrixSign block provides a way to adapt the texture of the plates connected to an overhang, based on Resource IDs of the texture files.
      |
      | For more information, please click Help.
      mask Help: eval('openHelp(733)')
      mask Display: image(imread('HighwaySpeedMatrix.png'))
  wires:
  VISUMatrixSign_HighwayOverhang_8/1 -> Actuator/1(VISUMatrixSign_HighwayOverhang_8)

== system TSR_Scenario_002_cs/VISUMatrixSign_HighwayOverhang_9 ==
  VISUMatrixSign_HighwayOverhang_9 : Inport  Tag=inport/VisuMatrixSign  SampleTime=1/100  BusOutputAsStruct=on
  Actuator : Subsystem  mask(PreScan Sink Block: VisuMatrixSign){UniqueID=875, ResourceList={'1' 'InformationSign\MatrixSign_GreenArrow.png' '2' 'InformationSign\Empty.jpeg' '3' 'InformationSign\SEARCH_Logo.png' '4' 'InformationSign\z274-50_black_full.png' '5' 'InformationSign\z274-51_black_full.png' '6' 'InformationSign\z274-52_black_full.png' '7' 'InformationSign\z274-53_black_full.png' '8' 'InformationSign\z274-54_black_full.png' '9' 'InformationSign\z274-55_black_full.png' '10' 'InformationSign\z274-56_black_full.png' '11' 'InformationSign\z274-57_black_full.png' '12' 'InformationSign\z274-58_black_full.png' '13' 'InformationSign\z274-59_black_full.png' '14' 'InformationSign\z274-60_black_full.png' '15' 'InformationSign\z274-61_black_full.png' '16' 'InformationSign\z274-62_black_full.png' '17' 'InformationSign\z274-63_black_full.png' }, PivotName=}
      mask prompts: UniqueID "Parent Unique Identifier (auto-generated)"; ResourceList "Resource List (auto-generated)"; PivotName "Name of pivot (auto-generated)"
      mask help:
      | The VisuMatrixSign block provides a way to adapt the texture of the plates connected to an overhang, based on Resource IDs of the texture files.
      |
      | For more information, please click Help.
      mask Help: eval('openHelp(733)')
      mask Display: image(imread('HighwaySpeedMatrix.png'))
  wires:
  VISUMatrixSign_HighwayOverhang_9/1 -> Actuator/1(VISUMatrixSign_HighwayOverhang_9)

== system TSR_Scenario_002_cs/WheelL0_Audi_A8_1 ==
  WheelL0_Audi_A8_1 : Inport  Tag=inport/JointActuator  OutDataTypeStr=Bus: PRESCAN_POSE_DATA  SampleTime=1/100  BusOutputAsStruct=on
  Actuator : Subsystem  Tag=VisuJoint  mask(PreScan Sink Block: VisuJoint){UniqueID=13, Translate_ObjectID3D=Audi_A8_1.WheelL0, Rotate_ObjectID3D=Audi_A8_1.WheelL0, TimeStep=1/100, DisplayName=[]}
      mask prompts: UniqueID "Parent Unique ID"; Translate_ObjectID3D "Translate Object Name"; Rotate_ObjectID3D "Rotate Object Name"; TimeStep "Simulation Step"; DisplayName "Display Name"
      mask help:
      | The VisuJoint block provides a way to adapt the location and orientation of a part of an object.
      |
      | For more information, please click Help.
      settings: DeleteFcn=PreScanBlockDeleteFcn;
      mask Help: eval('openHelp(223)')
      mask Display: image(imread('Joint.png'))
  wires:
  WheelL0_Audi_A8_1/1 -> Actuator/1(Joint)

== system TSR_Scenario_002_cs/WheelL0_BMW_X5_2 ==
  WheelL0_BMW_X5_2 : Inport  Tag=inport/JointActuator  OutDataTypeStr=Bus: PRESCAN_POSE_DATA  SampleTime=1/100  BusOutputAsStruct=on
  Actuator : Subsystem  Tag=VisuJoint  mask(PreScan Sink Block: VisuJoint){UniqueID=740, Translate_ObjectID3D=BMW_X5_2.WheelL0, Rotate_ObjectID3D=BMW_X5_2.WheelL0, TimeStep=1/100, DisplayName=[]}
      mask prompts: UniqueID "Parent Unique ID"; Translate_ObjectID3D "Translate Object Name"; Rotate_ObjectID3D "Rotate Object Name"; TimeStep "Simulation Step"; DisplayName "Display Name"
      mask help:
      | The VisuJoint block provides a way to adapt the location and orientation of a part of an object.
      |
      | For more information, please click Help.
      settings: DeleteFcn=PreScanBlockDeleteFcn;
      mask Help: eval('openHelp(223)')
      mask Display: image(imread('Joint.png'))
  wires:
  WheelL0_BMW_X5_2/1 -> Actuator/1(Joint)

== system TSR_Scenario_002_cs/WheelL0_Citroen_C3_1 ==
  WheelL0_Citroen_C3_1 : Inport  Tag=inport/JointActuator  OutDataTypeStr=Bus: PRESCAN_POSE_DATA  SampleTime=1/100  BusOutputAsStruct=on
  Actuator : Subsystem  Tag=VisuJoint  mask(PreScan Sink Block: VisuJoint){UniqueID=741, Translate_ObjectID3D=Citroen_C3_1.WheelL0, Rotate_ObjectID3D=Citroen_C3_1.WheelL0, TimeStep=1/100, DisplayName=[]}
      mask prompts: UniqueID "Parent Unique ID"; Translate_ObjectID3D "Translate Object Name"; Rotate_ObjectID3D "Rotate Object Name"; TimeStep "Simulation Step"; DisplayName "Display Name"
      mask help:
      | The VisuJoint block provides a way to adapt the location and orientation of a part of an object.
      |
      | For more information, please click Help.
      settings: DeleteFcn=PreScanBlockDeleteFcn;
      mask Help: eval('openHelp(223)')
      mask Display: image(imread('Joint.png'))
  wires:
  WheelL0_Citroen_C3_1/1 -> Actuator/1(Joint)

== system TSR_Scenario_002_cs/WheelL0_Fiat_Bravo_1 ==
  WheelL0_Fiat_Bravo_1 : Inport  Tag=inport/JointActuator  OutDataTypeStr=Bus: PRESCAN_POSE_DATA  SampleTime=1/100  BusOutputAsStruct=on
  Actuator : Subsystem  Tag=VisuJoint  mask(PreScan Sink Block: VisuJoint){UniqueID=742, Translate_ObjectID3D=Fiat_Bravo_1.WheelL0, Rotate_ObjectID3D=Fiat_Bravo_1.WheelL0, TimeStep=1/100, DisplayName=[]}
      mask prompts: UniqueID "Parent Unique ID"; Translate_ObjectID3D "Translate Object Name"; Rotate_ObjectID3D "Rotate Object Name"; TimeStep "Simulation Step"; DisplayName "Display Name"
      mask help:
      | The VisuJoint block provides a way to adapt the location and orientation of a part of an object.
      |
      | For more information, please click Help.
      settings: DeleteFcn=PreScanBlockDeleteFcn;
      mask Help: eval('openHelp(223)')
      mask Display: image(imread('Joint.png'))
  wires:
  WheelL0_Fiat_Bravo_1/1 -> Actuator/1(Joint)

== system TSR_Scenario_002_cs/WheelL0_Nissan_Cabstar_1 ==
  WheelL0_Nissan_Cabstar_1 : Inport  Tag=inport/JointActuator  OutDataTypeStr=Bus: PRESCAN_POSE_DATA  SampleTime=1/100  BusOutputAsStruct=on
  Actuator : Subsystem  Tag=VisuJoint  mask(PreScan Sink Block: VisuJoint){UniqueID=729, Translate_ObjectID3D=Nissan_Cabstar_1.WheelL0, Rotate_ObjectID3D=Nissan_Cabstar_1.WheelL0, TimeStep=1/100, DisplayName=[]}
      mask prompts: UniqueID "Parent Unique ID"; Translate_ObjectID3D "Translate Object Name"; Rotate_ObjectID3D "Rotate Object Name"; TimeStep "Simulation Step"; DisplayName "Display Name"
      mask help:
      | The VisuJoint block provides a way to adapt the location and orientation of a part of an object.
      |
      | For more information, please click Help.
      settings: DeleteFcn=PreScanBlockDeleteFcn;
      mask Help: eval('openHelp(223)')
      mask Display: image(imread('Joint.png'))
  wires:
  WheelL0_Nissan_Cabstar_1/1 -> Actuator/1(Joint)

== system TSR_Scenario_002_cs/WheelL1_Audi_A8_1 ==
  WheelL1_Audi_A8_1 : Inport  Tag=inport/JointActuator  OutDataTypeStr=Bus: PRESCAN_POSE_DATA  SampleTime=1/100  BusOutputAsStruct=on
  Actuator : Subsystem  Tag=VisuJoint  mask(PreScan Sink Block: VisuJoint){UniqueID=13, Translate_ObjectID3D=Audi_A8_1.WheelL1, Rotate_ObjectID3D=Audi_A8_1.WheelL1, TimeStep=1/100, DisplayName=[]}
      mask prompts: UniqueID "Parent Unique ID"; Translate_ObjectID3D "Translate Object Name"; Rotate_ObjectID3D "Rotate Object Name"; TimeStep "Simulation Step"; DisplayName "Display Name"
      mask help:
      | The VisuJoint block provides a way to adapt the location and orientation of a part of an object.
      |
      | For more information, please click Help.
      settings: DeleteFcn=PreScanBlockDeleteFcn;
      mask Help: eval('openHelp(223)')
      mask Display: image(imread('Joint.png'))
  wires:
  WheelL1_Audi_A8_1/1 -> Actuator/1(Joint)

== system TSR_Scenario_002_cs/WheelL1_BMW_X5_2 ==
  WheelL1_BMW_X5_2 : Inport  Tag=inport/JointActuator  OutDataTypeStr=Bus: PRESCAN_POSE_DATA  SampleTime=1/100  BusOutputAsStruct=on
  Actuator : Subsystem  Tag=VisuJoint  mask(PreScan Sink Block: VisuJoint){UniqueID=740, Translate_ObjectID3D=BMW_X5_2.WheelL1, Rotate_ObjectID3D=BMW_X5_2.WheelL1, TimeStep=1/100, DisplayName=[]}
      mask prompts: UniqueID "Parent Unique ID"; Translate_ObjectID3D "Translate Object Name"; Rotate_ObjectID3D "Rotate Object Name"; TimeStep "Simulation Step"; DisplayName "Display Name"
      mask help:
      | The VisuJoint block provides a way to adapt the location and orientation of a part of an object.
      |
      | For more information, please click Help.
      settings: DeleteFcn=PreScanBlockDeleteFcn;
      mask Help: eval('openHelp(223)')
      mask Display: image(imread('Joint.png'))
  wires:
  WheelL1_BMW_X5_2/1 -> Actuator/1(Joint)

== system TSR_Scenario_002_cs/WheelL1_Citroen_C3_1 ==
  WheelL1_Citroen_C3_1 : Inport  Tag=inport/JointActuator  OutDataTypeStr=Bus: PRESCAN_POSE_DATA  SampleTime=1/100  BusOutputAsStruct=on
  Actuator : Subsystem  Tag=VisuJoint  mask(PreScan Sink Block: VisuJoint){UniqueID=741, Translate_ObjectID3D=Citroen_C3_1.WheelL1, Rotate_ObjectID3D=Citroen_C3_1.WheelL1, TimeStep=1/100, DisplayName=[]}
      mask prompts: UniqueID "Parent Unique ID"; Translate_ObjectID3D "Translate Object Name"; Rotate_ObjectID3D "Rotate Object Name"; TimeStep "Simulation Step"; DisplayName "Display Name"
      mask help:
      | The VisuJoint block provides a way to adapt the location and orientation of a part of an object.
      |
      | For more information, please click Help.
      settings: DeleteFcn=PreScanBlockDeleteFcn;
      mask Help: eval('openHelp(223)')
      mask Display: image(imread('Joint.png'))
  wires:
  WheelL1_Citroen_C3_1/1 -> Actuator/1(Joint)

== system TSR_Scenario_002_cs/WheelL1_Fiat_Bravo_1 ==
  WheelL1_Fiat_Bravo_1 : Inport  Tag=inport/JointActuator  OutDataTypeStr=Bus: PRESCAN_POSE_DATA  SampleTime=1/100  BusOutputAsStruct=on
  Actuator : Subsystem  Tag=VisuJoint  mask(PreScan Sink Block: VisuJoint){UniqueID=742, Translate_ObjectID3D=Fiat_Bravo_1.WheelL1, Rotate_ObjectID3D=Fiat_Bravo_1.WheelL1, TimeStep=1/100, DisplayName=[]}
      mask prompts: UniqueID "Parent Unique ID"; Translate_ObjectID3D "Translate Object Name"; Rotate_ObjectID3D "Rotate Object Name"; TimeStep "Simulation Step"; DisplayName "Display Name"
      mask help:
      | The VisuJoint block provides a way to adapt the location and orientation of a part of an object.
      |
      | For more information, please click Help.
      settings: DeleteFcn=PreScanBlockDeleteFcn;
      mask Help: eval('openHelp(223)')
      mask Display: image(imread('Joint.png'))
  wires:
  WheelL1_Fiat_Bravo_1/1 -> Actuator/1(Joint)

== system TSR_Scenario_002_cs/WheelL1_Nissan_Cabstar_1 ==
  WheelL1_Nissan_Cabstar_1 : Inport  Tag=inport/JointActuator  OutDataTypeStr=Bus: PRESCAN_POSE_DATA  SampleTime=1/100  BusOutputAsStruct=on
  Actuator : Subsystem  Tag=VisuJoint  mask(PreScan Sink Block: VisuJoint){UniqueID=729, Translate_ObjectID3D=Nissan_Cabstar_1.WheelL1, Rotate_ObjectID3D=Nissan_Cabstar_1.WheelL1, TimeStep=1/100, DisplayName=[]}
      mask prompts: UniqueID "Parent Unique ID"; Translate_ObjectID3D "Translate Object Name"; Rotate_ObjectID3D "Rotate Object Name"; TimeStep "Simulation Step"; DisplayName "Display Name"
      mask help:
      | The VisuJoint block provides a way to adapt the location and orientation of a part of an object.
      |
      | For more information, please click Help.
      settings: DeleteFcn=PreScanBlockDeleteFcn;
      mask Help: eval('openHelp(223)')
      mask Display: image(imread('Joint.png'))
  wires:
  WheelL1_Nissan_Cabstar_1/1 -> Actuator/1(Joint)
